simulink library "trs"  (Simulink 8.1)
settings: Solver=ode1  StartTime=0.0  StopTime=Inf  FixedStep=0.001  RelTol=1e-3
PostLoadFcn:
  | , if any(exist('dsrtsu_mdlpostloadfcn', 'file') == [2, 3, 6]), try dsrtsu_mdlpostloadfcn('Execute', bdroot); catch fprintf('Error in PostLoadFcn (dsrtsu_mdlpostloadfcn) for model "%s":\n %s\n', bdroot, lasterr); end, end,
undefined symbols (not defined in the file or in its folder): C_TICK_TIME_S, KACC_TqCalcOverrideRollAvgInterval_s, KACC_TqCalcRollAvgInterval_s
libraries: hcu_lib x1
settings Model: DSRTSU_INTERNAL_RTI_VER=450  DSRTSU_INTERNAL_RTI_TYPE=rti1401  RTICANMMDATA=struct('GeneralSetupData',struct('modelroot','D:\ELN150201_TAIWAN\trunk\AdasDragon\software\sw_development\arch\app\acc','generalsettings',struct('filesettings',struct('destfolder',struct('Name','RTICANMM_FILES','Check',1),'buildfolder',struct('Name','.','Check',1),'AbsDestfolder',struct('Name','D:\ELN150201_TAIWAN\trunk\AdasDragon\software\sw_development\arch\app\acc\RTICANMM_FILES'),'AbsBuildfolder',struct('Name','D:\ELN150201_TAIWAN\trunk\AdasDragon\software\sw_development\arch\app\acc'))),'options',struct('addpaths',1,'rmpaths',1,'addtrcexclusion',logical(1),'cannavigator',struct('checkmonitoring',0),'show_usrtrc',0,'use_usrtrc',0),'advanced',struct('options',[1 1 1 1 1 1 1 1 1 1 1 1 1 1 1 1 1 1 1 1 1 1 1 1 1 1 1 1 1 1 1 1 1 1 1 1 1 1 1 1 1 1 1 1 1 1 1 1 1 1 1 1 1 1 1 1 1 1 1 1 1 1 1 1 1 1 1 1 1 1 1 1 1 1 1 1 1 1 1 1 1 1 1 1 1 1 1 1 1 1 1 1 1 1 1 1 1 1 1 1]),'MPSetup',{{}},'modelname','trs','block','trs'))  DSRTSU_INTERNAL_RTIFPGA=40  Creator=AT015411  LastModifiedBy=AT015555

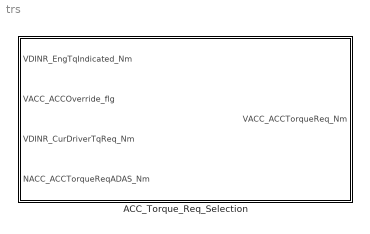
== system trs ==
  ACC_Torque_Req_Selection : Subsystem

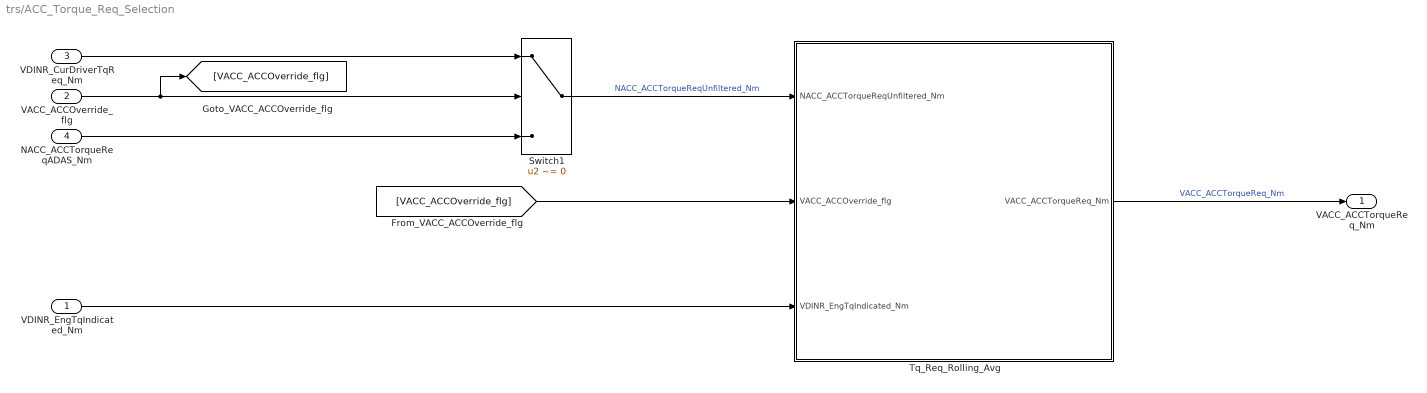
== system trs/ACC_Torque_Req_Selection ==
  VDINR_EngTqIndicated_Nm : Inport
  VACC_ACCOverride_flg : Inport  Port=2
  VDINR_CurDriverTqReq_Nm : Inport  Port=3
  NACC_ACCTorqueReqADAS_Nm : Inport  Port=4
  Switch1 : Switch  Criteria=u2 ~= 0
  Tq_Req_Rolling_Avg : Subsystem
  VACC_ACCTorqueReq_Nm : Outport
  wires:
  NACC_ACCTorqueReqADAS_Nm/1 -> Switch1/3
  VDINR_CurDriverTqReq_Nm/1 -> Switch1/1
  VACC_ACCOverride_flg/1 -> [VACC_ACCOverride_flg], Switch1/2
  Tq_Req_Rolling_Avg/1(VACC_ACCTorqueReq_Nm) -> VACC_ACCTorqueReq_Nm/1  "VACC_ACCTorqueReq_Nm"
  Switch1/1 -> Tq_Req_Rolling_Avg/1(NACC_ACCTorqueReqUnfiltered_Nm)  "NACC_ACCTorqueReqUnfiltered_Nm"
  VDINR_EngTqIndicated_Nm/1 -> Tq_Req_Rolling_Avg/3(VDINR_EngTqIndicated_Nm)
  [VACC_ACCOverride_flg] -> Tq_Req_Rolling_Avg/2(VACC_ACCOverride_flg)

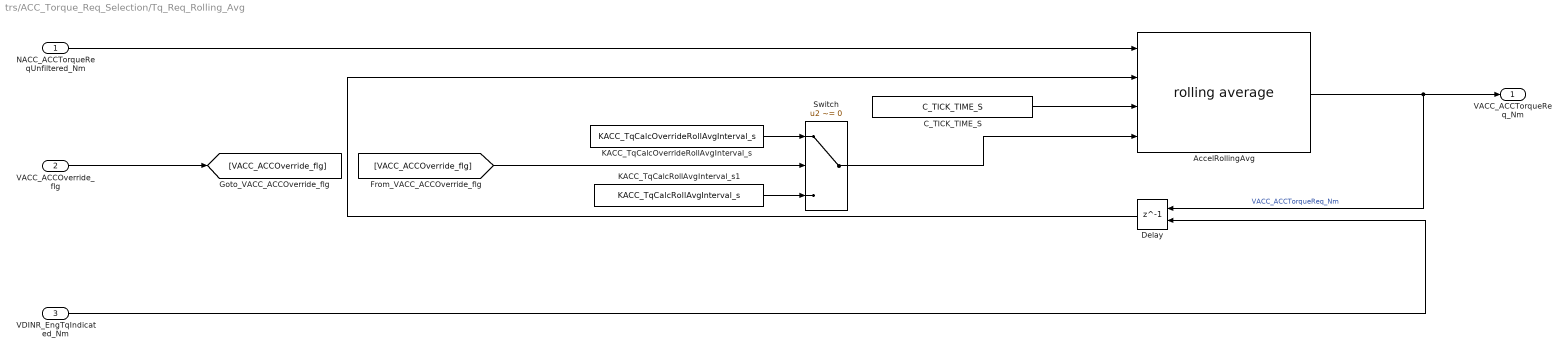
== system trs/ACC_Torque_Req_Selection/Tq_Req_Rolling_Avg ==
  NACC_ACCTorqueReqUnfiltered_Nm : Inport
  VACC_ACCOverride_flg : Inport  Port=2
  VDINR_EngTqIndicated_Nm : Inport  Port=3
  AccelRollingAvg : hcu_lib/rolling average
  C_TICK_TIME_S : Constant  Value=C_TICK_TIME_S
  Delay : Delay  DelayLength=1  InitialConditionSource=Input port
      settings: InputPortMap=u0,p4
  KACC_TqCalcOverrideRollAvgInterval_s : Constant  Value=KACC_TqCalcOverrideRollAvgInterval_s
  KACC_TqCalcRollAvgInterval_s1 : Constant  Value=KACC_TqCalcRollAvgInterval_s
  Switch : Switch  Criteria=u2 ~= 0
  VACC_ACCTorqueReq_Nm : Outport
  wires:
  Delay/1 -> AccelRollingAvg/2
  AccelRollingAvg/1 -> VACC_ACCTorqueReq_Nm/1, Delay/1  "VACC_ACCTorqueReq_Nm"
  C_TICK_TIME_S/1 -> AccelRollingAvg/3
  NACC_ACCTorqueReqUnfiltered_Nm/1 -> AccelRollingAvg/1
  KACC_TqCalcRollAvgInterval_s1/1 -> Switch/3
  KACC_TqCalcOverrideRollAvgInterval_s/1 -> Switch/1
  Switch/1 -> AccelRollingAvg/4
  VDINR_EngTqIndicated_Nm/1 -> Delay/2
  VACC_ACCOverride_flg/1 -> [VACC_ACCOverride_flg]
  [VACC_ACCOverride_flg] -> Switch/2
